simulink model "Nomoto_simulink"  (R2020a)
settings: Solver=VariableStepAuto  StartTime=0.0  StopTime=500  RelTol=1e-3
values from neighbouring files (symbols this model uses):
  A = [0, 1 ... (first row only)    [Nomoto.m]
  B = [0 ... (first row only)    [Nomoto.m]
  C = eye(2)    [Nomoto.m]
libraries: simulink x2
settings Model: Creator=micro microndas  LastModifiedBy=micro microndas

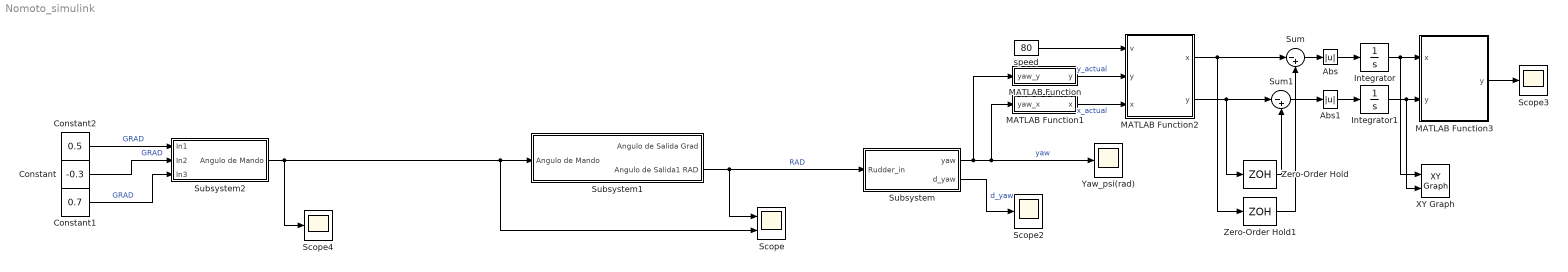
== system Nomoto_simulink ==
  Abs : Abs
  Abs1 : Abs
  Constant : Constant  Value=-0.3
  Constant1 : Constant  Value=0.7
  Constant2 : Constant  Value=0.5
  Integrator : Integrator
  Integrator1 : Integrator
  MATLAB Function : MATLAB Function  TreatAsAtomicUnit=on
  MATLAB Function1 : MATLAB Function  TreatAsAtomicUnit=on
  MATLAB Function2 : MATLAB Function  TreatAsAtomicUnit=on
  MATLAB Function3 : MATLAB Function  TreatAsAtomicUnit=on
  Scope : Scope  NumInputPorts=2
  Scope2 : Scope
  Scope3 : Scope
  Scope4 : Scope
  Subsystem : Subsystem
  Subsystem1 : Subsystem
  Subsystem2 : Subsystem
  Sum : Sum  Inputs=|-+
  Sum1 : Sum  Inputs=|-+
  XY Graph : simulink/Sinks/XY Graph  xmin=-20  xmax=20  ymin=-20  ymax=20  st=0.1
  Yaw_psi(rad) : Scope
  Zero-Order Hold : ZeroOrderHold  SampleTime=-1
  Zero-Order Hold1 : ZeroOrderHold  SampleTime=-1
  speed : Constant  Value=80
  wires:
  Subsystem1/2(Angulo de Salida1 RAD) -> Subsystem/1(Rudder_in), Scope/1  "RAD"
  Subsystem2/1(Angulo de Mando) -> Scope/2, Subsystem1/1(Angulo de Mando), Scope4/1
  Subsystem/1(yaw) -> MATLAB Function/1(yaw_y), MATLAB Function1/1(yaw_x), Yaw_psi(rad)/1  "yaw"
  Subsystem/2(d_yaw) -> Scope2/1  "d_yaw"
  MATLAB Function/1(y) -> MATLAB Function2/2("y ")  "y_actual"
  MATLAB Function1/1(x) -> MATLAB Function2/3("x ")  "x_actual"
  speed/1 -> MATLAB Function2/1(v)
  MATLAB Function2/1(x) -> Zero-Order Hold1/1, Sum/1
  MATLAB Function2/2(y) -> Zero-Order Hold/1, Sum1/1
  Zero-Order Hold/1 -> Sum1/2
  Zero-Order Hold1/1 -> Sum/2
  Integrator/1 -> XY Graph/1, MATLAB Function3/1(x)
  Integrator1/1 -> XY Graph/2, MATLAB Function3/2("y ")
  MATLAB Function3/1(y) -> Scope3/1
  Constant2/1 -> Subsystem2/1(In1)  "GRAD"
  Constant/1 -> Subsystem2/2(In2)  "GRAD"
  Constant1/1 -> Subsystem2/3(In3)  "GRAD"
  Sum1/1 -> Abs1/1
  Abs1/1 -> Integrator1/1
  Sum/1 -> Abs/1
  Abs/1 -> Integrator/1

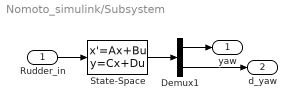
== system Nomoto_simulink/Subsystem ==
  Rudder_in : Inport
  Demux1 : Demux  Outputs=2
  State-Space : StateSpace  A=A  B=B  C=C  D=[0;0]  InitialCondition=0  ContinuousStateAttributes={'yaw','d_yaw'}
  yaw : Outport
  d_yaw : Outport  Port=2
  wires:
  Rudder_in/1 -> State-Space/1
  State-Space/1 -> Demux1/1
  Demux1/1 -> yaw/1
  Demux1/2 -> d_yaw/1

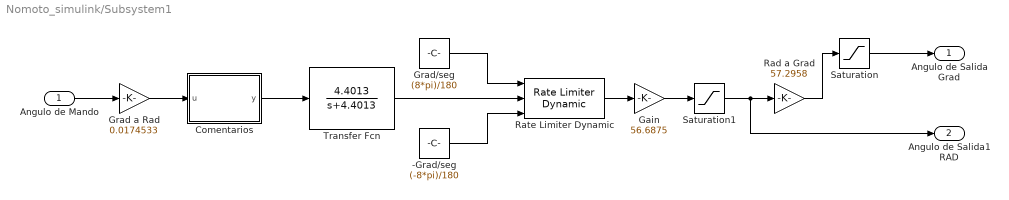
== system Nomoto_simulink/Subsystem1 ==
  Angulo de Mando : Inport
  -Grad/seg : Constant  Value=(-8*pi)/180
  Comentarios : MATLAB Function  TreatAsAtomicUnit=on
  Gain : Gain  Gain=56.6875
  Grad a Rad : Gain  Gain=0.0174533
  Grad/seg : Constant  Value=(8*pi)/180
  Rad a Grad : Gain  Gain=57.2958
  Rate Limiter Dynamic : simulink/Discontinuities/Rate Limiter Dynamic
  Saturation : Saturate
  Saturation1 : Saturate  UpperLimit=1.5  LowerLimit=-1.5
  Transfer Fcn : TransferFcn  Numerator=[4.4013]  Denominator=[1 4.4013]
  Angulo de Salida Grad : Outport
  Angulo de Salida1 RAD : Outport  Port=2
  wires:
  Transfer Fcn/1 -> Rate Limiter Dynamic/2
  Grad/seg/1 -> Rate Limiter Dynamic/1
  -Grad/seg/1 -> Rate Limiter Dynamic/3
  Comentarios/1(y) -> Transfer Fcn/1
  Rad a Grad/1 -> Saturation/1
  Saturation/1 -> Angulo de Salida Grad/1
  Rate Limiter Dynamic/1 -> Gain/1
  Grad a Rad/1 -> Comentarios/1(u)
  Angulo de Mando/1 -> Grad a Rad/1
  Saturation1/1 -> Angulo de Salida1 RAD/1, Rad a Grad/1
  Gain/1 -> Saturation1/1

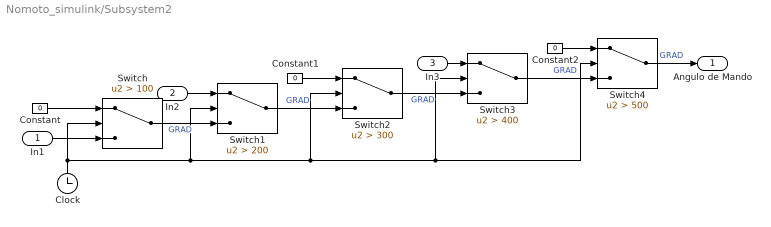
== system Nomoto_simulink/Subsystem2 ==
  In1 : Inport
  In2 : Inport  Port=2
  In3 : Inport  Port=3
  Clock : Clock
  Constant : Constant  Value=0
  Constant1 : Constant  Value=0
  Constant2 : Constant  Value=0
  Switch : Switch  Criteria=u2 > Threshold  Threshold=100
  Switch1 : Switch  Criteria=u2 > Threshold  Threshold=200
  Switch2 : Switch  Criteria=u2 > Threshold  Threshold=300
  Switch3 : Switch  Criteria=u2 > Threshold  Threshold=400
  Switch4 : Switch  Criteria=u2 > Threshold  Threshold=500
  Angulo de Mando : Outport
  wires:
  Clock/1 -> Switch1/2, Switch2/2, Switch3/2, Switch4/2, Switch/2
  In1/1 -> Switch/3
  Constant/1 -> Switch/1
  Switch/1 -> Switch1/3  "GRAD"
  In2/1 -> Switch1/1
  Switch1/1 -> Switch2/3  "GRAD"
  Constant1/1 -> Switch2/1
  Switch2/1 -> Switch3/3  "GRAD"
  In3/1 -> Switch3/1
  Switch3/1 -> Switch4/3  "GRAD"
  Constant2/1 -> Switch4/1
  Switch4/1 -> Angulo de Mando/1  "GRAD"

== matlab function Nomoto_simulink/MATLAB Function ==
  data: yaw_y input; y output
function y = fcn(yaw_y)

y = sin(yaw_y);

== matlab function Nomoto_simulink/Subsystem1/Comentarios ==
  data: u input; y output
function y = fcn(u)

%Kg' = Kg*L / U
    %Kg = Maximo giro del timon / error maximo
        %error maximo
        %Maximo giro del timon
    %L = Eslora / Longitud del buque
        %390.00 𝑓𝑡 
        %118.872 mts
    %U = Velocidad del buque
        %15 nudo nautico
        %7.7166 m/s

y = u;

== matlab function Nomoto_simulink/MATLAB Function1 ==
  data: yaw_x input; x output
function x = fcn(yaw_x)

x = cos(yaw_x);

== matlab function Nomoto_simulink/MATLAB Function2 ==
  data: x output; v input; y output; y input; x input
function [x,y] = fcn(v,y,x)
x = v*x;
y = v*y;

== matlab function Nomoto_simulink/MATLAB Function3 ==
  data: x input; y output; y input
function y = fcn(x,y)

y = atan(y/x);
